simulink model "CRCL"  (R2020b)
settings: Solver=FixedStepDiscrete  StartTime=0.0  StopTime=inf  FixedStep=0.01  RelTol=1e-3  EnableMultiTasking=on
values from neighbouring files (symbols this model uses):
  calibrationDelayTime_s = 2.0    [CRCL_Dictionary.sldd]
  collisionAngleThreshold_deg = 40.0    [CRCL_Dictionary.sldd]
  collisionVarianceThreshold_g2 = 8.0    [CRCL_Dictionary.sldd]
  cpMaxAbortTime_s = 30.0    [CRCL_Dictionary.sldd]
  cpMaxTipOverAngle_deg = 35.0    [CRCL_Dictionary.sldd]
  cpMinEstDistance_m = 50.0    [CRCL_Dictionary.sldd]
  cpMinEstDistanceGnssBased_m = 200.0    [CRCL_Dictionary.sldd]
  cpMinRiddenTime_s = 15.0    [CRCL_Dictionary.sldd]
  cpMinSpeedRiding_kmh = 10.0    [CRCL_Dictionary.sldd]
  cpNumCrankRevolutionThreshold = 5.0    [CRCL_Dictionary.sldd]
  cpSpeedCond2PositiveSpeedChangeTime_s = 5.0    [CRCL_Dictionary.sldd]
  cpSpeedDerivativeThreshold_kmhs = 0.005    [CRCL_Dictionary.sldd]
  cpTimeOutSpeedCond2_s = 15.0    [CRCL_Dictionary.sldd]
  groundHitEnergyThresholdStanding_g2s2 = 0.02    [CRCL_Dictionary.sldd]
  groundHitTipOverAngleThreshold_deg = 40.0    [CRCL_Dictionary.sldd]
  longAccCompForEulerEstFlag = 0.0    [CRCL_Dictionary.sldd]
  minEnergyStrongHit_g2s2 = 0.1    [CRCL_Dictionary.sldd]
  noMotionAccVarianceThresholdSD_g2 = 0.001    [CRCL_Dictionary.sldd]
  ride1minSpeedSlow_kmh = 4.0    [CRCL_Dictionary.sldd]
  ride2minSpeed_kmh = 8.0    [CRCL_Dictionary.sldd]
  rroMaxSpeed_kmh = 5.0    [CRCL_Dictionary.sldd]
  rroMinGyrX_degs = 20.0    [CRCL_Dictionary.sldd]
  rroMonotonyThreshold_degs = -1.0    [CRCL_Dictionary.sldd]
  rroRollIntegrationAngleThreshold_degs = 20.0    [CRCL_Dictionary.sldd]
  rroUniContinuityThreshold_degs = 15.0    [CRCL_Dictionary.sldd]
  scaleFactorVarianceStrongHit = 2.0    [CRCL_Dictionary.sldd]
  sdoMaxAccVarFreeFall_g2 = 0.06    [CRCL_Dictionary.sldd]
  sdoMaxTipOverAngle_deg = 20.0    [CRCL_Dictionary.sldd]
  sdoMinAccVar_g2 = 8.0    [CRCL_Dictionary.sldd]
  sdoMinGyrXYNorm_degs = 720.0    [CRCL_Dictionary.sldd]
  sdoMinGyrXYNormFreeFall_degs = 100.0    [CRCL_Dictionary.sldd]
  sdoMinOrientationChange_deg = 120.0    [CRCL_Dictionary.sldd]
  sdoScaleFactorOrientationChange = 3.0    [CRCL_Dictionary.sldd]
  stepTime_s = 0.01    [CRCL_Dictionary.sldd]
  strongHitSafetyFactor = 2.5    [CRCL_Dictionary.sldd]
  tipOverAccZFiltTreshold_g = 0.7    [CRCL_Dictionary.sldd]
  tipOverAngleThreshold_deg = 50.0    [CRCL_Dictionary.sldd]
  tipOverMinAccZFiltNoseOver_g = 0.3    [CRCL_Dictionary.sldd]
  tipOverRollPitchRelationNoseOver = 1.5    [CRCL_Dictionary.sldd]
undefined symbols (not defined in the file or in its folder): magnitude
libraries: simulink x17
(part 4 of 8)

== stateflow chart CRCL/RideDetection_RD ==
  state Init
    en:
    RD_RIDE_TIMEOUT = single(5); %sec
    RD_fire = int16(0);
  state NoRide
    en:
    RD_fire = int16(0);
  state PossibleRideFast
  state RideFast
    %RD -> 2
  state Ride
    %RD -> 1
  note: Überprüfung TipOver nur am Anfang???, besser kontinuierlich!!!
  state Latch
    en:
    %check if speed drop has been caused by hubConnection loss
    if ~(RD_hubConnection == 0 && ...
    RD_systemConfig == 2 && RD_cobiHubSetup ~= 1)
    RD_fire = int16(1);
    end
  RideFast -> Ride [order 2] : %[RD_curSpeed < RD_minSpeed || ...
      | %(RD_curSpeed <= 13 && RD_curSpeedDerivative <= -2.5)]
      | [RD_curSpeed < RD_minSpeed || ...
      | (RD_curSpeed <= 16 && RD_curSpeedDerivative <= -2.5 && RD_curSpeedDerivative <= (-0.5*RD_curSpeed+4))]
      |
      | {
      | RD_fire = int16(1);
      | }
  (default) -> Init
  Init -> NoRide
  PossibleRideFast -> Ride [order 1] : [RD_curSpeed < RD_minSpeed]
      | {
      | RD_fire = int16(1);
      | }
  PossibleRideFast -> RideFast [order 2] : [after(2,sec)]
      | {
      | RD_fire = int16(2);
      | }
  NoRide -> Ride : %[(RD_curSpeed >= RD_minSpeed) && (TO_fire ==0)]
      | [RD_curSpeed >= RD_minSpeedSlow]
      | {
      | RD_fire = int16(1);
      | }
  Ride -> PossibleRideFast [order 1] : [RD_curSpeed >= RD_minSpeed]
  RideFast -> Latch [order 1] : [RD_curSpeed < RD_minSpeedSlow]
  Latch -> Ride [order 2] : [RD_curSpeed > RD_minSpeedSlow]
  Ride -> Latch [order 2] : [RD_curSpeed < RD_minSpeedSlow]
  Latch -> NoRide [order 1] : [after(RD_RIDE_TIMEOUT, sec)]
      | {
      |
      | }
  data: RD_curSpeed input; RD_fire output; RD_RIDE_TIMEOUT local; RD_curSpeedDerivative input; RD_minSpeedSlow input; RD_minSpeed input; RD_hubConnection input; RD_systemConfig input; RD_cobiHubSetup input
